simulink model "pendulum_control"  (R2022b)
settings: Solver=VariableStepAuto  StartTime=0.0  StopTime=8  MaxStep=.02  RelTol=1e-3
values from neighbouring files (symbols this model uses):
  A = [0,1,0,0;0,0,-(m*g)/M,0;0,0,0,1;0,0,(m+M)*g/(M*L),0]    [Run_Me.m]
  B = [0;1/M;0;-1/(M*L)]    [Run_Me.m]
  Ctf = tf(ss(u_x_ss.A-L1*u_x_ss.C-u_x_ss.B*K1, L1, K1, 0))    [Run_Me.m]
  g = 9.81    [Run_Me.m]
  K = place(A, B, [-1 -1.5 -2 -2.5]-2)    [Run_Me.m]    (also in partial_state_feedback.m = place(sys2_ss.A, sys2_ss.B, [-2 -3 -4]))
  K1 = place(u_x_ss.A, u_x_ss.B, [-1 -2 -3 -4])    [Run_Me.m]
  L = 1    [Run_Me.m]
  L1 = place(u_x_ss.A.', u_x_ss.C.', [-1 -2 -3 -4]-10).'    [Run_Me.m]
  m = .1    (= 0.1)    [Run_Me.m]
  M = 1    [Run_Me.m]
  u_x_ss = ss(u_x_tf)    [Run_Me.m]
  u_x_tf = sys_tf(1)    [Run_Me.m]
settings Model: Creator=hp_desktop  LastModifiedBy=hp_desktop

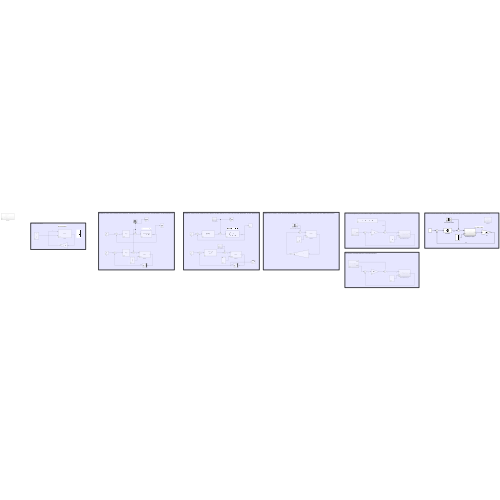
[thumbnail: Simulink's stored preview of the top-level diagram]
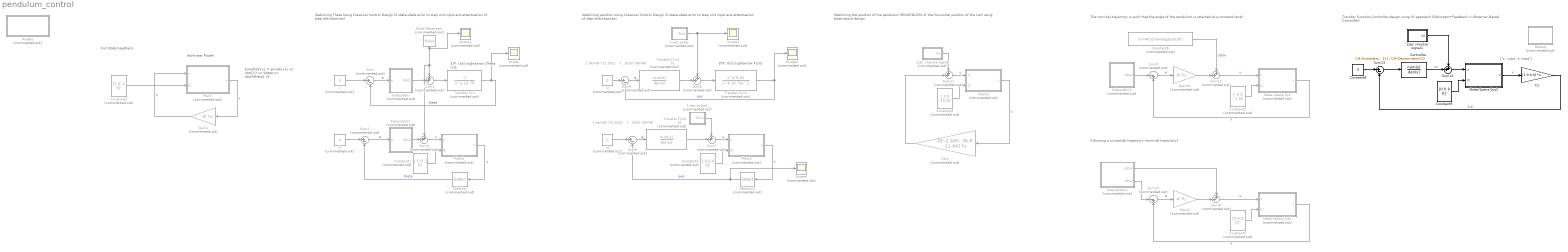
== system pendulum_control ==
  note: Stabilizing Theta Using Classical Control Design (0 state-state error to step unit input and attentuation of step disturbances)
  note: Full State Feedback
  note: $TF: U(s) \rightarrow \Theta (s)$
  note: Nonlinear Model
  note: $\mathbf{x} = \pmatrix{x \cr \dot{x} \cr \theta \cr \dot{\theta} }$
  note: Stabilizing position Using Classical Control Design (0 state-state error to step unit input and attentuation of step disturbances)
  note: $TF: U(s) \rightarrow X(s)$
  note: Stabilizing the position of the pendulum REGARDLESS of the horizontal position of the cart using state-space design.
  note: The nominal trajectory is such that the angle of the pendulum is retained at a constant level!
  note: Following a sinusoidal trajectory (nominal trajectory)
  note: Transfer Function Controller design using SS approach (Estimator+Feedback = Observer-Based Controller)
  note: {'x','xdot','t','tdot'}
  1-sec pulse : Subsystem  Commented=on
  1-sec pulse1 : Subsystem  Commented=on
  1sec impulse signal : Subsystem  Commented=on  mask{impulse_magnitude=2.5, impulse_time=3}
      mask prompts: impulse_magnitude "Magnitude"; impulse_time "Time"
      mask Display: plot([0 4 4 5 5 10], [0 0 1 1 0 0]);
  1sec impulse signal1 : Subsystem  mask{impulse_magnitude=.1, impulse_time=1, impulse_interval=0.2}
      mask prompts: impulse_magnitude "Magnitude"; impulse_time "Time"; impulse_interval "Interval of Impulse"
      mask Display: plot([0 4 4 5 5 10], [0 0 1 1 0 0]);
  C1 : Gain  Gain=[1 0 0 0]  Multiplication=Matrix(K*u)
  Constant1 : Constant  Commented=on  Value=[.5 0 .1 0]'  VectorParams1D=off
  Constant2 : Constant  Commented=on  Value=[1 0 .1 0]'  VectorParams1D=off
  Constant3 : Constant  Commented=on  Value=[.0 0 0 0]'  VectorParams1D=off
  Constant4 : Constant  Commented=on  Value=[.2 0 .15 0]'  VectorParams1D=off
  Constant5 : Constant  Commented=on  Value=[-.5 0 -.1 0]'  VectorParams1D=off
  Constant6 : Constant  Commented=on  Value=(m+M)*g*tan(deg2rad(10))
  Constant7 : Constant  Commented=on  Value=[0 0 0 0]'  VectorParams1D=off
  Constant8 : Constant  Value=0
  Constant9 : Constant  Value=[0 0 0 0]'  VectorParams1D=off
  Controller : TransferFcn  Numerator=Ctf.Numerator{1}  Denominator=Ctf.Denominator{1}
  Details : Subsystem  Commented=on
  Gain : Gain  Commented=on  Gain=-[0 -2.445 -36.8 -11.44]  Multiplication=Matrix(K*u)
  Gain1 : Gain  Commented=on  Gain=-K  Multiplication=Matrix(K*u)
  Gain10 : Gain  Commented=on  Gain=-K  Multiplication=Matrix(K*u)
  Gain2 : Gain  Commented=on  Gain=-K  Multiplication=Matrix(K*u)
  Models : Subsystem  Commented=on
  Plant : Subsystem  Commented=on
      mask Display: disp('Plant');
  Plant1 : Subsystem  Commented=on
      mask Display: disp('Plant');
  Plant2 : Subsystem  Commented=on
      mask Display: disp('Plant');
  Plant3 : Subsystem  Commented=on
      mask Display: disp('Plant');
  Pulse Generator : DiscretePulseGenerator  Commented=on  PulseType=Time based  Amplitude=20  Period=10  PulseWidth=2  PhaseDelay=5
  Scope{,1..4} (5 alike) : Scope  Commented=on
  Selector : Selector  Commented=on  InputPortWidth=4  IndexOptions=Index vector (dialog)  Indices=3  OutputSizes=1
  Selector1 : Selector  Commented=on  InputPortWidth=4  IndexOptions=Index vector (dialog)  Indices=1  OutputSizes=1
  State-Space Sys : Subsystem  Commented=on
  State-Space Sys1 : Subsystem  Commented=on
  State-Space Sys2 : Subsystem
  Subsystem : Subsystem  Commented=on
      mask Display: disp('C(s)');
  Subsystem1 : Subsystem  Commented=on
      mask Display: disp('C(s)');
  Subsystem2 : Subsystem  Commented=on
  Subsystem4 : Subsystem  Commented=on
  Sum{,2,4,6} (4 alike) : Sum  Commented=on  Inputs=|+-
  Sum{1,3,5,7..8,11..12} (7 alike) : Sum  Commented=on  Inputs=++|
  Sum10 : Sum  Commented=on  Inputs=|-+
  Sum13 : Sum  Inputs=|+-
  Sum14 : Sum  Inputs=++|
  Sum9 : Sum  Commented=on  Inputs=|-+
  Transfer Fcn : TransferFcn  Commented=on  Numerator=-1  Denominator=[1 0 -10.79]
  Transfer Fcn1 : TransferFcn  Commented=on  Numerator=[1 0 -9.81]  Denominator=[1 0 -10.79 0 0]
  Transfer Fcn2 : TransferFcn  Commented=on  Numerator="1.0e+08 * [2.2022    7.1788   -0.2132   -0.1114   -0.0270]"  Denominator="[1          949.269413946124          450545.419126812         -213617423.786385         -673460193.706748                         0]"
  Transfer Fcn3 : TransferFcn  Commented=on  Numerator="1.0e+08 * [2.2022    7.1788   -0.2132   -0.1114   -0.0270]"  Denominator="[1          949.269413946124          450545.419126812         -213617423.786385         -673460193.706748                         0]"
  r{,1..3} (4 alike) : Constant  Commented=on  Value=0
  wires:
  Constant2/1 -> Plant/2(IC)
  Gain1/1 -> Plant/1(u)  "u"
  Plant/1(x) -> Gain1/1  "x"
  Subsystem/1(Out1) -> Sum1/2
  Sum/1 -> Subsystem/1(e)  "e"
  Transfer Fcn/1 -> Scope/1, Sum/2  "theta"
  r/1 -> Sum/1
  Sum1/1 -> Transfer Fcn/1
  Subsystem1/1(Out1) -> Sum3/2
  Plant1/1(x) -> Selector/1  "x"
  r1/1 -> Sum2/1
  Selector/1 -> Sum2/2  "theta"
  Sum2/1 -> Subsystem1/1(e)  "e"
  Constant1/1 -> Plant1/2(IC)
  Sum3/1 -> Plant1/1(u)  "u"
  Pulse Generator/1 -> Scope1/1, Sum3/1, Sum1/1
  Sum7/1 -> Plant2/1(u)  "u"
  Constant3/1 -> Plant2/2(IC)
  Sum6/1 -> Transfer Fcn2/1  "e"
  Selector1/1 -> Scope4/1, Sum6/2  "pos"
  r3/1 -> Sum6/1
  Plant2/1(x) -> Selector1/1  "x"
  Transfer Fcn2/1 -> Sum7/2
  Sum5/1 -> Transfer Fcn1/1
  r2/1 -> Sum4/1
  Transfer Fcn1/1 -> Scope2/1, Sum4/2  "pos"
  Sum4/1 -> Transfer Fcn3/1  "e"
  Transfer Fcn3/1 -> Sum5/2
  1-sec pulse/1(Out1) -> Scope3/1, Sum5/1
  1-sec pulse1/1(Out1) -> Sum7/1
  Plant3/1(x) -> Gain/1  "x"
  Constant4/1 -> Plant3/2(IC)
  Sum11/1 -> Plant3/1(u)  "u"
  Gain/1 -> Sum11/2
  1sec impulse signal/1(du) -> Sum11/1
  Constant5/1 -> State-Space Sys/2(IC)
  State-Space Sys/1(x) -> Sum9/2  "x"
  Constant6/1 -> Sum12/1  "uStar"
  Sum12/1 -> State-Space Sys/1(u)  "u"
  Sum9/1 -> Gain10/1  "e"
  Gain10/1 -> Sum12/2
  Subsystem2/1(xStar) -> Sum9/1
  Subsystem4/2(xStar) -> Sum10/1
  Gain2/1 -> Sum8/2
  Sum10/1 -> Gain2/1  "e"
  Sum8/1 -> State-Space Sys1/1(u)  "u"
  State-Space Sys1/1(x) -> Sum10/2  "x"
  Constant7/1 -> State-Space Sys1/2(IC)
  Subsystem4/1(uStar) -> Sum8/1
  Sum14/1 -> State-Space Sys2/1(u)
  C1/1 -> Sum13/2  "Y(s)"
  1sec impulse signal1/1(du) -> Sum14/1
  Constant9/1 -> State-Space Sys2/2(IC)
  Sum13/1 -> Controller/1
  Controller/1 -> Sum14/2  "uc"
  Constant8/1 -> Sum13/1
  State-Space Sys2/1(x) -> C1/1  "x"

== system pendulum_control/1-sec pulse ==
  Step : Step  Time=3  SampleTime=0
  Step1 : Step  Time=4  After=-1  SampleTime=0
  Sum8 : Sum
  Out1 : Outport
  wires:
  Step1/1 -> Sum8/2
  Step/1 -> Sum8/1
  Sum8/1 -> Out1/1

== system pendulum_control/1-sec pulse1 ==
  Step : Step  Time=3  After=.02  SampleTime=0
  Step1 : Step  Time=4  After=-.02  SampleTime=0
  Sum8 : Sum
  Out1 : Outport
  wires:
  Sum8/1 -> Out1/1
  Step/1 -> Sum8/1
  Step1/1 -> Sum8/2

== system pendulum_control/1sec impulse signal ==
  Step : Step  Time=impulse_time  After=impulse_magnitude  SampleTime=0
  Step1 : Step  Time=impulse_time+1  After=-impulse_magnitude  SampleTime=0
  Sum8 : Sum
  du : Outport
  wires:
  Step1/1 -> Sum8/2
  Step/1 -> Sum8/1
  Sum8/1 -> du/1

== system pendulum_control/1sec impulse signal1 ==
  Step : Step  Time=impulse_time  After=impulse_magnitude  SampleTime=0
  Step1 : Step  Time=impulse_time+impulse_interval  After=-impulse_magnitude  SampleTime=0
  Sum8 : Sum
  du : Outport
  wires:
  Sum8/1 -> du/1
  Step/1 -> Sum8/1
  Step1/1 -> Sum8/2

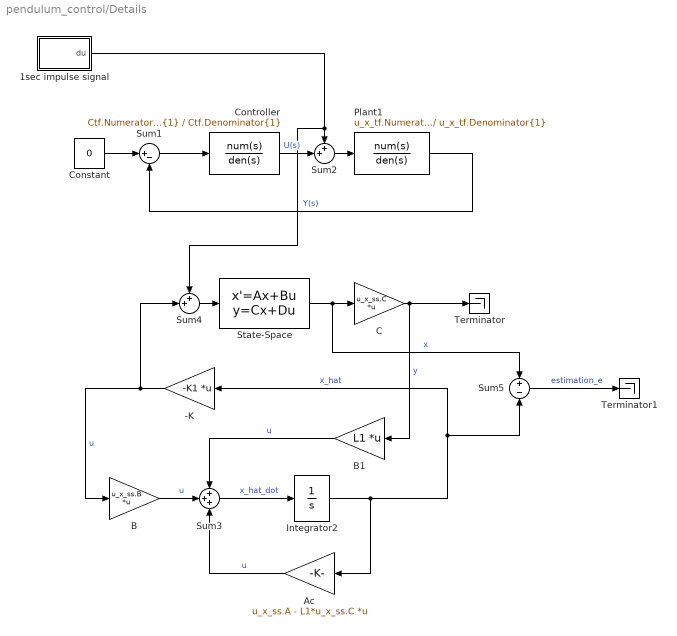
== system pendulum_control/Details ==
  -K : Gain  Gain=-K1  Multiplication=Matrix(K*u)
  1sec impulse signal : Subsystem  mask{impulse_magnitude=.1, impulse_time=1, impulse_interval=0.2}
      mask prompts: impulse_magnitude "Magnitude"; impulse_time "Time"; impulse_interval "Interval of Impulse"
      mask Display: plot([0 4 4 5 5 10], [0 0 1 1 0 0]);
  Ac : Gain  Gain=u_x_ss.A - L1*u_x_ss.C  Multiplication=Matrix(K*u)
  B : Gain  Gain=u_x_ss.B  Multiplication=Matrix(K*u)
  B1 : Gain  Gain=L1  Multiplication=Matrix(K*u)
  C : Gain  Gain=u_x_ss.C  Multiplication=Matrix(K*u)
  Constant : Constant  Value=0
  Controller : TransferFcn  Numerator=Ctf.Numerator{1}  Denominator=Ctf.Denominator{1}
  Integrator2 : Integrator
  Plant1 : TransferFcn  Numerator=u_x_tf.Numerator{1}  Denominator=u_x_tf.Denominator{1}
  State-Space : StateSpace  A=u_x_ss.A  B=u_x_ss.B  C=eye(4)  D=[0 0 0 0]'  InitialCondition=[0 0 0 0]
  Sum1 : Sum  Inputs=|+-
  Sum2 : Sum  Inputs=++|
  Sum3 : Sum  Inputs=+++
  Sum4 : Sum  Inputs=++|
  Sum5 : Sum  Inputs=+|-
  Terminator : Terminator
  Terminator1 : Terminator
  wires:
  B1/1 -> Sum3/1  "u"
  Integrator2/1 -> Sum5/2, -K/1, Ac/1  "x_hat"
  B/1 -> Sum3/2  "u"
  Sum5/1 -> Terminator1/1  "estimation_e"
  State-Space/1 -> Sum5/1, C/1  "x"
  -K/1 -> B/1, Sum4/2  "u"
  C/1 -> B1/1, Terminator/1  "y"
  Controller/1 -> Sum2/2  "U(s)"
  Plant1/1 -> Sum1/2  "Y(s)"
  Sum4/1 -> State-Space/1
  Sum2/1 -> Plant1/1
  Sum1/1 -> Controller/1
  1sec impulse signal/1(du) -> Sum4/1, Sum2/1
  Sum3/1 -> Integrator2/1  "x_hat_dot"
  Constant/1 -> Sum1/1
  Ac/1 -> Sum3/3  "u"

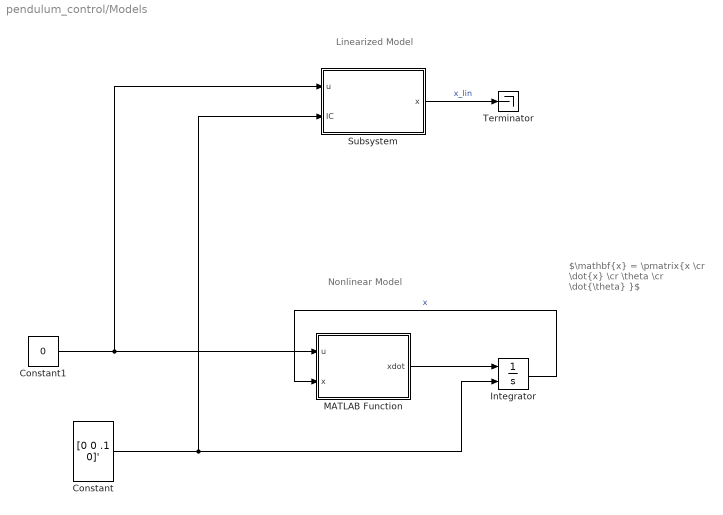
== system pendulum_control/Models ==
  note: Linearized Model
  note: Nonlinear Model
  note: $\mathbf{x} = \pmatrix{x \cr \dot{x} \cr \theta \cr \dot{\theta} }$
  Constant : Constant  Value=[0 0 .1 0]'  VectorParams1D=off
  Constant1 : Constant  Value=0
  Integrator : Integrator  InitialConditionSource=external
  MATLAB Function : MATLAB Function  TreatAsAtomicUnit=on
  Subsystem : Subsystem
  Terminator : Terminator
  wires:
  Constant1/1 -> Subsystem/1(u), MATLAB Function/1(u)
  Subsystem/1(x) -> Terminator/1  "x_lin"
  Integrator/1 -> MATLAB Function/2(x)  "x"
  Constant/1 -> Subsystem/2(IC), Integrator/2
  MATLAB Function/1(xdot) -> Integrator/1

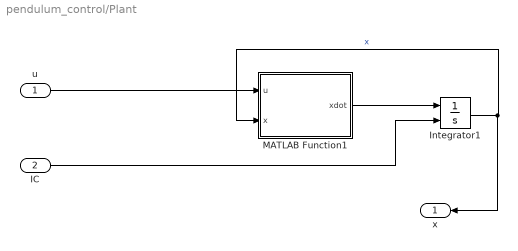
== system pendulum_control/Plant ==
  u : Inport
  IC : Inport  Port=2
  Integrator1 : Integrator  InitialConditionSource=external
  MATLAB Function1 : MATLAB Function  TreatAsAtomicUnit=on
  x : Outport
  wires:
  Integrator1/1 -> x/1, MATLAB Function1/2(x)  "x"
  u/1 -> MATLAB Function1/1(u)
  MATLAB Function1/1(xdot) -> Integrator1/1
  IC/1 -> Integrator1/2

== system pendulum_control/Plant1 ==
  u : Inport
  IC : Inport  Port=2
  Integrator1 : Integrator  InitialConditionSource=external
  MATLAB Function1 : MATLAB Function  TreatAsAtomicUnit=on
  x : Outport
  wires:
  IC/1 -> Integrator1/2
  MATLAB Function1/1(xdot) -> Integrator1/1
  u/1 -> MATLAB Function1/1(u)
  Integrator1/1 -> MATLAB Function1/2(x), x/1  "x"

== system pendulum_control/Plant2 ==
  u : Inport
  IC : Inport  Port=2
  Integrator1 : Integrator  InitialConditionSource=external
  MATLAB Function1 : MATLAB Function  TreatAsAtomicUnit=on
  x : Outport
  wires:
  Integrator1/1 -> x/1, MATLAB Function1/2(x)  "x"
  u/1 -> MATLAB Function1/1(u)
  MATLAB Function1/1(xdot) -> Integrator1/1
  IC/1 -> Integrator1/2

== system pendulum_control/Plant3 ==
  u : Inport
  IC : Inport  Port=2
  Integrator1 : Integrator  InitialConditionSource=external
  MATLAB Function1 : MATLAB Function  TreatAsAtomicUnit=on
  x : Outport
  wires:
  IC/1 -> Integrator1/2
  MATLAB Function1/1(xdot) -> Integrator1/1
  u/1 -> MATLAB Function1/1(u)
  Integrator1/1 -> MATLAB Function1/2(x), x/1  "x"

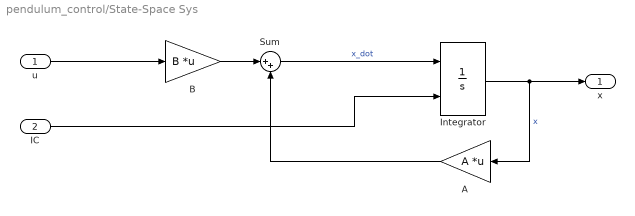
== system pendulum_control/State-Space Sys ==
  u : Inport
  IC : Inport  Port=2
  A : Gain  Gain=A  Multiplication=Matrix(K*u)
  B : Gain  Gain=B  Multiplication=Matrix(K*u)
  Integrator : Integrator  InitialConditionSource=external  ContinuousStateAttributes={'x','xdot','t','tdot'}
  Sum : Sum  Inputs=|++
  x : Outport
  wires:
  B/1 -> Sum/1
  Integrator/1 -> x/1, A/1  "x"
  Sum/1 -> Integrator/1  "x_dot"
  IC/1 -> Integrator/2
  A/1 -> Sum/2
  u/1 -> B/1

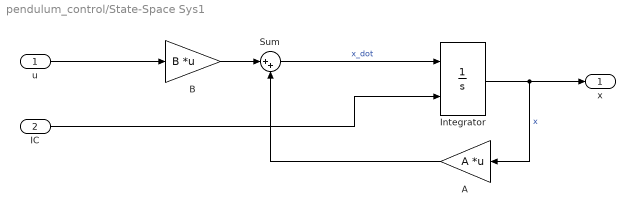
== system pendulum_control/State-Space Sys1 ==
  u : Inport
  IC : Inport  Port=2
  A : Gain  Gain=A  Multiplication=Matrix(K*u)
  B : Gain  Gain=B  Multiplication=Matrix(K*u)
  Integrator : Integrator  InitialConditionSource=external  ContinuousStateAttributes={'x','xdot','t','tdot'}
  Sum : Sum  Inputs=|++
  x : Outport
  wires:
  u/1 -> B/1
  A/1 -> Sum/2
  IC/1 -> Integrator/2
  Sum/1 -> Integrator/1  "x_dot"
  Integrator/1 -> A/1, x/1  "x"
  B/1 -> Sum/1

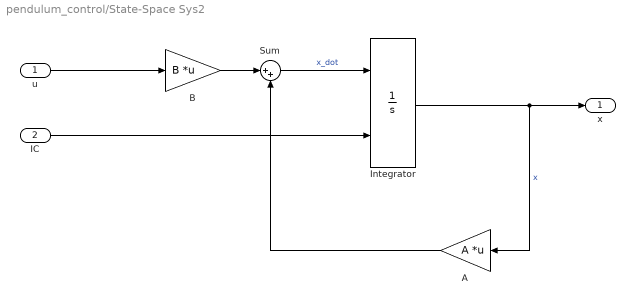
== system pendulum_control/State-Space Sys2 ==
  u : Inport
  IC : Inport  Port=2
  A : Gain  Gain=A  Multiplication=Matrix(K*u)
  B : Gain  Gain=B  Multiplication=Matrix(K*u)
  Integrator : Integrator  InitialConditionSource=external  ContinuousStateAttributes={'x','xdot','t','tdot'}
  Sum : Sum  Inputs=|++
  x : Outport
  wires:
  u/1 -> B/1
  A/1 -> Sum/2
  IC/1 -> Integrator/2
  Sum/1 -> Integrator/1  "x_dot"
  Integrator/1 -> A/1, x/1  "x"
  B/1 -> Sum/1

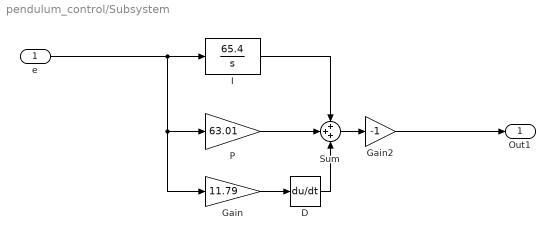
== system pendulum_control/Subsystem ==
  e : Inport
  D : Derivative
  Gain : Gain  Gain=11.79
  Gain2 : Gain  Gain=-1
  I : TransferFcn  Numerator=65.4  Denominator=[1 0]
  P : Gain  Gain=63.01
  Sum : Sum  Inputs=+++
  Out1 : Outport
  wires:
  Gain/1 -> D/1
  D/1 -> Sum/3
  e/1 -> Gain/1, P/1, I/1
  Sum/1 -> Gain2/1
  P/1 -> Sum/2
  I/1 -> Sum/1
  Gain2/1 -> Out1/1

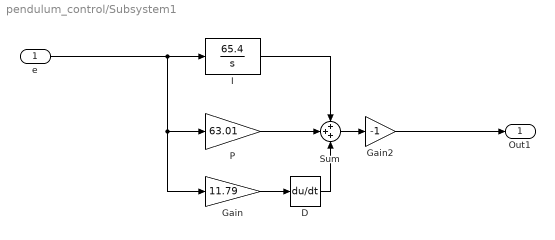
== system pendulum_control/Subsystem1 ==
  e : Inport
  D : Derivative
  Gain : Gain  Gain=11.79
  Gain2 : Gain  Gain=-1
  I : TransferFcn  Numerator=65.4  Denominator=[1 0]
  P : Gain  Gain=63.01
  Sum : Sum  Inputs=+++
  Out1 : Outport
  wires:
  Gain2/1 -> Out1/1
  I/1 -> Sum/1
  P/1 -> Sum/2
  Sum/1 -> Gain2/1
  e/1 -> I/1, P/1, Gain/1
  D/1 -> Sum/3
  Gain/1 -> D/1

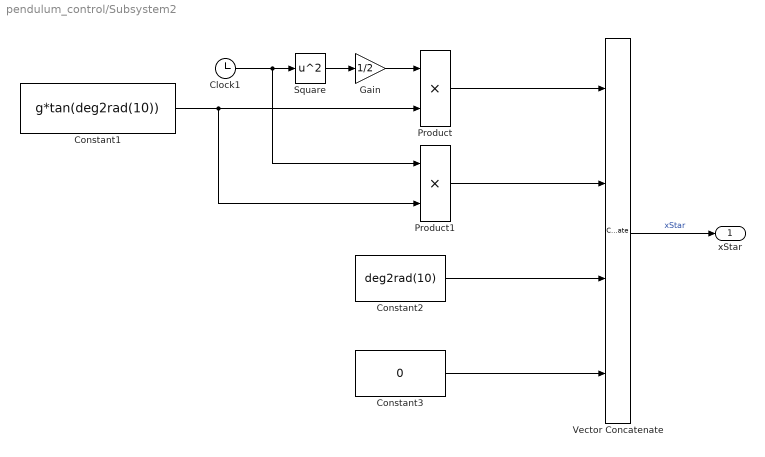
== system pendulum_control/Subsystem2 ==
  Clock1 : Clock
  Constant1 : Constant  Value=g*tan(deg2rad(10))
  Constant2 : Constant  Value=deg2rad(10)
  Constant3 : Constant  Value=0
  Gain : Gain  Gain=1/2
  Product : Product
  Product1 : Product
  Square : Math  Operator=square
  Vector Concatenate : Concatenate  NumInputs=4
  xStar : Outport
  wires:
  Vector Concatenate/1 -> xStar/1  "xStar"
  Product/1 -> Vector Concatenate/1
  Clock1/1 -> Product1/1, Square/1
  Square/1 -> Gain/1
  Constant1/1 -> Product1/2, Product/2
  Gain/1 -> Product/1
  Product1/1 -> Vector Concatenate/2
  Constant2/1 -> Vector Concatenate/3
  Constant3/1 -> Vector Concatenate/4

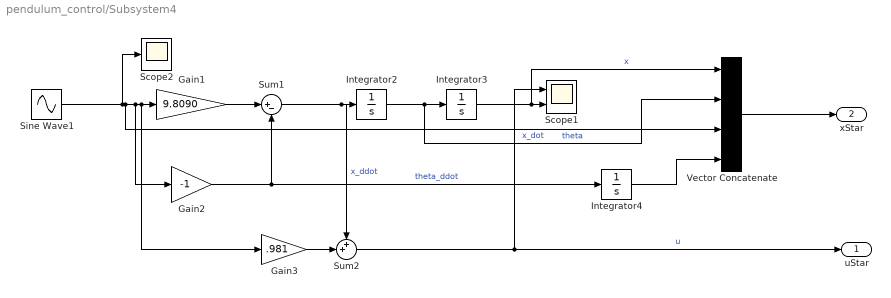
== system pendulum_control/Subsystem4 ==
  Gain1 : Gain  Gain=9.8090
  Gain2 : Gain  Gain=-1
  Gain3 : Gain  Gain=.981
  Integrator2 : Integrator
  Integrator3 : Integrator
  Integrator4 : Integrator
  Scope1 : Scope  NumInputPorts=2
  Scope2 : Scope
  Sine Wave1 : Sin  Amplitude=.25  Frequency=2  Phase=pi/2  SampleTime=0
  Sum1 : Sum  Inputs=|+-
  Sum2 : Sum  Inputs=++|
  Vector Concatenate : Concatenate  NumInputs=4
  uStar : Outport
  xStar : Outport  Port=2
  wires:
  Sine Wave1/1 -> Scope2/1, Vector Concatenate/3, Gain2/1, Gain3/1, Gain1/1  "theta"
  Gain2/1 -> Integrator4/1, Sum1/2  "theta_ddot"
  Sum2/1 -> uStar/1, Scope1/1  "u"
  Gain3/1 -> Sum2/2
  Integrator2/1 -> Vector Concatenate/2, Integrator3/1  "x_dot"
  Integrator3/1 -> Vector Concatenate/1, Scope1/2  "x"
  Gain1/1 -> Sum1/1
  Sum1/1 -> Sum2/1, Integrator2/1  "x_ddot"
  Vector Concatenate/1 -> xStar/1
  Integrator4/1 -> Vector Concatenate/4

== system pendulum_control/Details/1sec impulse signal ==
  Step : Step  Time=impulse_time  After=impulse_magnitude  SampleTime=0
  Step1 : Step  Time=impulse_time+impulse_interval  After=-impulse_magnitude  SampleTime=0
  Sum8 : Sum
  du : Outport
  wires:
  Step1/1 -> Sum8/2
  Step/1 -> Sum8/1
  Sum8/1 -> du/1

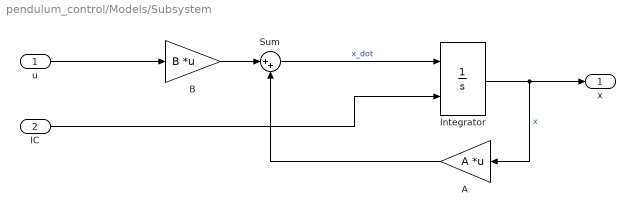
== system pendulum_control/Models/Subsystem ==
  u : Inport
  IC : Inport  Port=2
  A : Gain  Gain=A  Multiplication=Matrix(K*u)
  B : Gain  Gain=B  Multiplication=Matrix(K*u)
  Integrator : Integrator  InitialConditionSource=external  ContinuousStateAttributes={'x','xdot','t','tdot'}
  Sum : Sum  Inputs=|++
  x : Outport
  wires:
  B/1 -> Sum/1
  Integrator/1 -> x/1, A/1  "x"
  Sum/1 -> Integrator/1  "x_dot"
  IC/1 -> Integrator/2
  A/1 -> Sum/2
  u/1 -> B/1

== matlab function pendulum_control/Plant/MATLAB Function1 ==
  data: u input; xdot output; x input; g parameter; L parameter; m parameter; M parameter
function xdot = fcn(u, x, g, L, m, M)

% x_ = x(1);
% xdot_ = x(2);
t = x(3);
tdot = x(4);

% M*qddot + c = [u;0] where q = [x, theta]'

Q = [m+M,m*L*cos(t);m*L*cos(t),m*L^2];
c = [-m*L*tdot^2*sin(t);-m*g*L*sin(t)];
qddot = Q\(-c+[u;0]);

xdot = [x(2); qddot(1); x(4); qddot(2)];

== matlab function pendulum_control/Models/MATLAB Function ==
  data: u input; xdot output; x input; g parameter; L parameter; m parameter; M parameter
function xdot = fcn(u, x, g, L, m, M)

% x_ = x(1);
% xdot_ = x(2);
t = x(3);
tdot = x(4);

% M*qddot + c = [u;0] where q = [x, theta]'

Q = [m+M,m*L*cos(t);m*L*cos(t),m*L^2];
c = [-m*L*tdot^2*sin(t);-m*g*L*sin(t)];
qddot = Q\(-c+[u;0]);

xdot = [x(2); qddot(1); x(4); qddot(2)];

== matlab function pendulum_control/Plant1/MATLAB Function1 ==
  data: u input; xdot output; x input; g parameter; L parameter; m parameter; M parameter
function xdot = fcn(u, x, g, L, m, M)

% x_ = x(1);
% xdot_ = x(2);
t = x(3);
tdot = x(4);

% M*qddot + c = [u;0] where q = [x, theta]'

Q = [m+M,m*L*cos(t);m*L*cos(t),m*L^2];
c = [-m*L*tdot^2*sin(t);-m*g*L*sin(t)];
qddot = Q\(-c+[u;0]);

xdot = [x(2); qddot(1); x(4); qddot(2)];

== matlab function pendulum_control/Plant2/MATLAB Function1 ==
  data: u input; xdot output; x input; g parameter; L parameter; m parameter; M parameter
function xdot = fcn(u, x, g, L, m, M)

% x_ = x(1);
% xdot_ = x(2);
t = x(3);
tdot = x(4);

% M*qddot + c = [u;0] where q = [x, theta]'

Q = [m+M,m*L*cos(t);m*L*cos(t),m*L^2];
c = [-m*L*tdot^2*sin(t);-m*g*L*sin(t)];
qddot = Q\(-c+[u;0]);

xdot = [x(2); qddot(1); x(4); qddot(2)];

== matlab function pendulum_control/Plant3/MATLAB Function1 ==
  data: u input; xdot output; x input; g parameter; L parameter; m parameter; M parameter
function xdot = fcn(u, x, g, L, m, M)

% x_ = x(1);
% xdot_ = x(2);
t = x(3);
tdot = x(4);

% M*qddot + c = [u;0] where q = [x, theta]'

Q = [m+M,m*L*cos(t);m*L*cos(t),m*L^2];
c = [-m*L*tdot^2*sin(t);-m*g*L*sin(t)];
qddot = Q\(-c+[u;0]);

xdot = [x(2); qddot(1); x(4); qddot(2)];
